simulink library "vmc"  (R2021b)
settings: Solver=VariableStepAuto  StartTime=0.0  StopTime=10.0  RelTol=1e-3
undefined symbols (not defined in the file or in its folder): AVMC_ACCDeltaTqIGain4OVRD_X_kph, AVMC_ACCDeltaTqIGain4OVRD_Y_mps2, AVMC_ACCDeltaTqIGain_X_kph, AVMC_ACCDeltaTqIGain_Y_mps2, AVMC_ACCDeltaTqPGain_X_kph, AVMC_ACCDeltaTqPGain_Y_kph, AVMC_ACCLongSteadyCtrl_X_kph, AVMC_ADSPosGFBDeltaTq_X_kph, AVMC_ADSPosGFBDeltaTq_Y_mps2, AVMC_AggressJerkPCT4AT_X_kph, AVMC_AggressJerkPCT_X_kph, AVMC_AggressLimitPCT4AT_X_kph, AVMC_AggressLimitPCT_X_kph, AVMC_CCLongSteadyCtrl_X_kph, AVMC_DISCDeltaTqIGain_X_kph, AVMC_DISCDeltaTqIGain_Y_mps2, AVMC_DISCDeltaTqPGain_X_kph, AVMC_DISCDeltaTqPGain_Y_kph, AVMC_ESCRegenOut_X_kph, AVMC_ESCRegenOut_Y_Deg, AVMC_ESCRegenOutEnSpd_X_Deg, AVMC_ISOAccLimit_X_mps, AVMC_ISODecLimit_X_mps, AVMC_ISOJerk_X_mps, AVMC_LatESCRegenOut_X_kph, AVMC_LatESCRegenOut_Y_Deg, AVMC_LongAccDeadZone_X_kph, AVMC_LongAccFiltTsforP2_X_Gps, AVMC_MCPresBaseTq_X_bar, AVMC_MSALongSteadyCtrl_X_kph, AVMC_MSAPedalOvrd_X_kph, AVMC_MSASpdBand_X_kph, AVMC_MSATqDownEndTq_X_kph, AVMC_MSATqDownTime_X_kph, AVMC_OPDDisSlideRate_X_Deg, AVMC_OVRD2ActSR2FCMCMD_X_mps2, AVMC_PedalTqRWhlRatio_X_Nm, AVMC_PedalTqRWhlRatio_Y_gps, AVMC_PedalTqRWhlSlipGain_X_rat, AVMC_PedalTqRWhlSlipGain_Y_kph, AVMC_PedalTqRWhSTRGGain_X_deg, AVMC_PedalTqRWhSTRGGain_Y_kph, AVMC_RDCDetectTime_X_kph, AVMC_RDCDetectTime_Y_pct, AVMC_RDCEnSlideRate_X_Deg, AVMC_RearWhlTqRatio_X_Nm, AVMC_RearWhlTqRatio_Y_gps, AVMC_RearWhlTqSlipGain_X_rat, AVMC_RearWhlTqSlipGain_Y_kph, AVMC_RearWhlTqSTRGGain_X_deg, AVMC_RearWhlTqSTRGGain_Y_kph, AVMC_ReqBrkJoinDecSR_X_mps2, AVMC_SoftJerkPCT_X_kph, AVMC_SoftLimitPCT_X_kph, AVMC_StESCYaw_X_kph, AVMC_StESCYaw_Y_Deg, AVMC_StESCYawCom_X_kph, AVMC_StESCYawCom_Y_Gps, AVMC_TMSpdBaseTq_X_rpm, AVMC_VehHoldDecCtrlTime2_X_kph ... (+411)
libraries: hcu_lib x108, simulink x82, tqr x1, simulink_extras x1
(part 6 of 14)

== system vmc/VMC/VMC/ACC_Function/ACC Control Allow Judgement ==
  task_time_s : Inport
  VTQD_ExternalTqAllow_flag : Inport  Port=2
  VTQD_ExtDoorAllow_flg : Inport  Port=3
  AND : Logic  AllPortsSameDT=off  OutDataTypeStr=boolean
  Constant : Constant  Value=KVMC_ExternalTqAllowTime_s
  Constant3 : Constant  Value=TRUE
  Constant4 : Constant  Value=FALSE
  NOT : Logic  Operator=NOT  AllPortsSameDT=off  OutDataTypeStr=boolean
  Relational Operator : RelationalOperator  OutDataTypeStr=boolean  RndMeth=Simplest
  Timer : hcu_lib/Basic_Blocks/Timer
  u2>0 : Switch  Criteria=u2 > Threshold
  VVMC_ACCCtrlAllow_flg : Outport
  wires:
  task_time_s/1 -> [task_time_s]
  Constant/1 -> Relational Operator/2, Timer/4
  VTQD_ExternalTqAllow_flag/1 -> [VTQD_ExternalTqAllow_flag]
  NOT/1 -> Timer/2
  u2>0/1 -> [VVMC_ACCCtrlAllow_flg]  "VVMC_ACCCtrlAllow_flg"
  AND/1 -> NOT/1, Timer/1
  Constant4/1 -> u2>0/3
  Constant3/1 -> u2>0/1
  Timer/1 -> Relational Operator/1
  Relational Operator/1 -> u2>0/2
  [task_time_s] -> Timer/3
  [VVMC_ACCCtrlAllow_flg] -> VVMC_ACCCtrlAllow_flg/1
  [VTQD_ExtDoorAllow_flg] -> AND/2
  [VTQD_ExternalTqAllow_flag] -> AND/1
  VTQD_ExtDoorAllow_flg/1 -> [VTQD_ExtDoorAllow_flg]

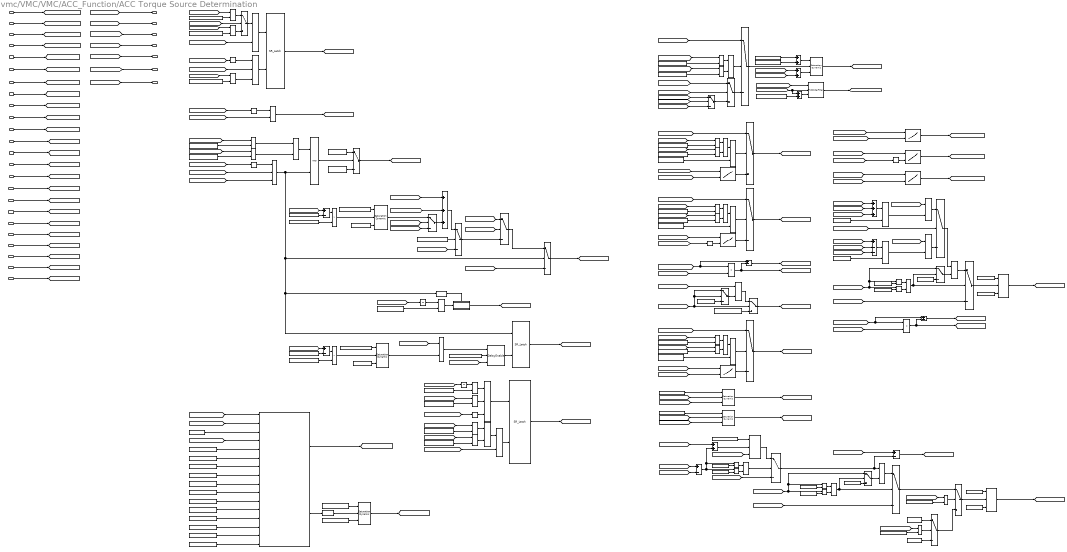
== system vmc/VMC/VMC/ACC_Function/ACC Torque Source Determination ==
  note: TRUE
  VTQD_DriverWhlTqDem_Nm : Inport
  VVMC_ADASWhlTqCal_Nm : Inport  Port=2
  VVMC_FeatArbitrFinal_enum : Inport  Port=3
  VTQD_LowIdleAccPedal_flg : Inport  Port=4
  VINP_ACCObjDist_m : Inport  Port=5
  VINP_TimeGapLevel_enum : Inport  Port=6
  VVMC_ADASActive_flg : Inport  Port=7
  task_time_s : Inport  Port=8
  VINP_LongAccel_Gps : Inport  Port=9
  VINP_VehSpeed_kph : Inport  Port=10
  VVMC_FrRrSlipSpd_kph : Inport  Port=11
  VVMC_CruzWhlTqReq_Nm : Inport  Port=12
  VVMC_CruzActive_flg : Inport  Port=13
  VVMC_MSAWhlTqReq_Nm : Inport  Port=14
  VVMC_MSAActive_flg : Inport  Port=15
  VTQD_RrEDUAvailBrkRgnTq_Nm : Inport  Port=16
  VTQD_FrEDUAvailBrkRgnTq_Nm : Inport  Port=17
  VPMM_DrivetrainSelect_enum : Inport  Port=18
  VINP_SASAngle_Deg : Inport  Port=19
  VDHP_ActAPSPosn_pct : Inport  Port=20
  VTQD_CreepBaseTqD_Nm : Inport  Port=21
  VVMC_ACCVehHoldReqRaw_flg : Inport  Port=22
  VVMC_ADASACCSta_enum : Inport  Port=23
  VTQD_EVDriveMode_enum : Inport  Port=24
  AND{,1,5..6,10,12} (6 alike) : Logic  AllPortsSameDT=off  OutDataTypeStr=boolean
  AND11 : Logic  Inputs=3  AllPortsSameDT=off  OutDataTypeStr=boolean
  AND{2..4,13} (4 alike) : Logic  Operator=OR  AllPortsSameDT=off  OutDataTypeStr=boolean
  Abs : Abs
  Abs1 : Abs
  Add{1,4..6,8,13} (6 alike) : Sum  Inputs=+-
  Add{9..11,28} (4 alike) : Sum
  Add2 : Sum  Inputs=+++
  Add3 : Sum  Inputs=+--
  Add7 : Sum  Inputs=+++
  Cast To Single : DataTypeConversion  OutDataTypeStr=single
  Constant1 : Constant  Value=FALSE
  Constant10 : Constant  Value=ENUM_TIMEGAPLEVEL_LEVEL1
  Constant11 : Constant  Value=ENUM_TIMEGAPLEVEL_LEVEL2
  Constant12 : Constant  Value=ENUM_TIMEGAPLEVEL_LEVEL3
  Constant13 : Constant  Value=ENUM_TIMEGAPLEVEL_LEVEL4
  Constant14 : Constant  Value=KVMC_TimeGapBandLv2_s
  Constant15 : Constant  Value=KVMC_TimeGapBandLv3_s
  Constant16 : Constant  Value=KVMC_TimeGapBandLv4_s
  Constant17 : Constant  Value=TRUE
  Constant18 : Constant  Value=FALSE
  Constant{19,24..26,39,41..46,48,50,52,57,59,65} (17 alike) : Constant  Value=ZERO_FLOAT
  Constant2 : Constant  Value=KTQD_AWDWhlTqRatioSW_flg
  Constant20 : Constant  Value=ENUM_DRIVEMODE_NRM
  Constant208 : Constant  Value=KVMC_ESCLongGBWFilter_raw32
  Constant21 : Constant  Value=KTQD_AWDWhlTqRatioSW_flg
  Constant22 : Constant  Value=ENUM_DRIVEMODE_NRM
  Constant23 : Constant  Value=ENUM_DRIVEMODE_SPORT
  Constant{27..28,37,40,49,51} (6 alike) : Constant  Value=ONE_FLOAT
  Constant29 : Constant  Value=ENUM_FEATARBITRSTA_ACC
  Constant3 : Constant  Value=TRUE
  Constant30 : Constant  Value=ENUM_FEATARBITRSTA_DISC
  Constant31 : Constant  Value=KTQD_RrUppTheldTrq_Nm
  Constant32 : Constant  Value=ENUM_DRIVETRAIN_AWD  VectorParams1D=off  SampleTime=-1
  Constant33 : Constant  Value=KTQD_RrUppTheldTrq_Nm
  Constant34 : Constant  Value=KTQD_RrUppTheldTrq_Nm
  Constant35 : Constant  Value=KTQD_FrUppTheldTrq_Nm
  Constant36 : Constant  Value=KTQD_FrUppTheldTrq_Nm
  Constant38 : Constant  Value=ENUM_DRIVETRAIN_RWD  VectorParams1D=off  SampleTime=-1
  Constant4 : Constant  Value=ENUM_FEATARBITRSTA_ACC
  Constant47 : Constant  Value=KVMC_TimeGapMax_s
  Constant5 : Constant  Value=ENUM_FEATARBITRSTA_DISC
  Constant53 : Constant  Value=KVMC_ACCPedalOvrdPosn_pct
  Constant54 : Constant  Value=KVMC_ACCPedalOvrdResPosn_pct
  Constant58 : Constant  Value=KVMC_ACCPedalOvrdPosn4Hold_pct
  Constant6 : Constant  Value=ENUM_DRIVEMODE_SPORT
  Constant62 : Constant  Value=KVMC_ACCOvrdTestSW_flg
  Constant63 : Constant  Value=KVMC_ACCPedalOvrdPosn_pct
  Constant64 : Constant  Value=KVMC_ACCOvrdPedalTqRatio_Nm
  Constant66 : Constant  Value=KVMC_ACCPedalOvrdRestTime_s
  Constant67 : Constant  Value=KVMC_ACCOvrdPedalTqLinearLim_Nm
  Constant68 : Constant  Value=KVMC_ACCPedalOvrdPosn_pct
  Constant69 : Constant  Value=KVMC_ACCOvrdPedalTqRatio_Nm
  Constant7 : Constant  Value=KVMC_TimeGapMax_s
  Constant71 : Constant  Value=ENUM_ADASACCSTA_STANDBY
  Constant72 : Constant  Value=ENUM_ADASACCSTA_ACTIVE
  Constant73 : Constant  Value=ENUM_ADASACCSTA_ACTIVE
  Constant74 : Constant  Value=ENUM_ADASACCSTA_OVERRIDE
  Constant75 : Constant  Value=KVMC_ACCOvrdPedalTqLinearLim_Nm
  Constant76 : Constant  Value=KTQD_AWDWhlTqRatioSW_flg
  Constant77 : Constant  Value=ENUM_DRIVEMODE_SPORT
  Constant78 : Constant  Value=ENUM_DRIVEMODE_NRM
  Constant8 : Constant  Value=KPH2MPS
  Constant9 : Constant  Value=KVMC_TimeGapBandLv1_s
  DelayEnable1 : hcu_lib/Basic_Blocks/DelayEnable
  Detect Increase : simulink/Logic and Bit Operations/Detect Increase  vinit=0.0  OutDataTypeStr=boolean
  Divide{,3,5,7} (4 alike) : Product  Inputs=**
  Divide1 : Product  Inputs=*/
  Divide2 : Product  Inputs=*/
  Divide4 : Product  Inputs=*/
  Equal{1..8} (8 alike) : RelationalOperator  Operator===  OutDataTypeStr=boolean  RndMeth=Simplest
  FirstOrderFilter6 : hcu_lib/Basic_Blocks/FirstOrderFilter
  Logical Operator1 : Logic  Inputs=3  AllPortsSameDT=off  OutDataTypeStr=boolean
  Logical Operator2 : Logic  Operator=OR  AllPortsSameDT=off  OutDataTypeStr=boolean
  Logical Operator4 : Logic  AllPortsSameDT=off  OutDataTypeStr=boolean
  Logical Operator5 : Logic  Operator=OR  AllPortsSameDT=off  OutDataTypeStr=boolean
  MMAP_PedalTqRWhlSlipGain_Z_Nm : Lookup_n-D  BreakpointsForDimension1=AVMC_PedalTqRWhlSlipGain_Y_kph  BreakpointsForDimension2=AVMC_PedalTqRWhlSlipGain_X_rat  Table=MVMC_PedalTqRWhlSlipGain_Z_Nm  InternalRulePriority=Speed  RndMeth=Simplest  InputSameDT=on
      settings: InputPortMap=u0,u1
  MMAP_RearWhlTqSlipGain_Z_Nm : Lookup_n-D  BreakpointsForDimension1=AVMC_RearWhlTqSlipGain_Y_kph  BreakpointsForDimension2=AVMC_RearWhlTqSlipGain_X_rat  Table=MVMC_RearWhlTqSlipGain_Z_Nm  InternalRulePriority=Speed  RndMeth=Simplest  InputSameDT=on
      settings: InputPortMap=u0,u1
  MVMC_PedalTqRWhSTRGGain_Z_Nm : Lookup_n-D  BreakpointsForDimension1=AVMC_PedalTqRWhSTRGGain_Y_kph  BreakpointsForDimension2=AVMC_PedalTqRWhSTRGGain_X_deg  Table=MVMC_PedalTqRWhSTRGGain_Z_Nm  InternalRulePriority=Speed  RndMeth=Simplest  InputSameDT=on
      settings: InputPortMap=u0,u1
  MVMC_PedalTqRWhlRatio_Z_rat : Lookup_n-D  BreakpointsForDimension1=AVMC_PedalTqRWhlRatio_Y_gps  BreakpointsForDimension2=AVMC_PedalTqRWhlRatio_X_Nm  Table=MVMC_PedalTqRWhlRatio_Z_rat  InternalRulePriority=Speed  RndMeth=Simplest  InputSameDT=on
      settings: InputPortMap=u0,u1
  MVMC_RearWhlTqRatio_Z_rat : Lookup_n-D  BreakpointsForDimension1=AVMC_RearWhlTqRatio_Y_gps  BreakpointsForDimension2=AVMC_RearWhlTqRatio_X_Nm  Table=MVMC_RearWhlTqRatio_Z_rat  InternalRulePriority=Speed  RndMeth=Simplest  InputSameDT=on
      settings: InputPortMap=u0,u1
  MVMC_RearWhlTqSTRGGain_Z_Nm : Lookup_n-D  BreakpointsForDimension1=AVMC_RearWhlTqSTRGGain_Y_kph  BreakpointsForDimension2=AVMC_RearWhlTqSTRGGain_X_deg  Table=MVMC_RearWhlTqSTRGGain_Z_Nm  InternalRulePriority=Speed  RndMeth=Simplest  InputSameDT=on
      settings: InputPortMap=u0,u1
  Max : MinMax  Function=max  Inputs=2
  Max1 : MinMax  Inputs=2
  Max2 : MinMax  Inputs=2
  Max3 : MinMax  Function=max  Inputs=2
  Min : MinMax  Function=max  Inputs=2
  NOT{,3,5,7} (4 alike) : Logic  Operator=NOT  AllPortsSameDT=off  OutDataTypeStr=boolean
  OR1 : Logic  Operator=OR  Inputs=3  AllPortsSameDT=off  OutDataTypeStr=boolean
  OR2 : Logic  Operator=OR  AllPortsSameDT=off  OutDataTypeStr=boolean
  OR3 : Logic  Operator=OR  AllPortsSameDT=off  OutDataTypeStr=boolean
  OR4 : Logic  Operator=OR  AllPortsSameDT=off  OutDataTypeStr=boolean
  Relational Operator{,11,13,19} (4 alike) : RelationalOperator  Operator=>  OutDataTypeStr=boolean  RndMeth=Simplest
  Relational Operator{10,12,14,16} (4 alike) : RelationalOperator  Operator=<  OutDataTypeStr=boolean  RndMeth=Simplest
  Relational Operator15 : RelationalOperator  OutDataTypeStr=boolean  RndMeth=Simplest
  Relational Operator17 : RelationalOperator  OutDataTypeStr=boolean  RndMeth=Simplest
  Relational Operator{2..3,5,9,21..22} (6 alike) : RelationalOperator  Operator===  OutDataTypeStr=boolean  RndMeth=Simplest
  Relational Operator23 : RelationalOperator  Operator=~=  OutDataTypeStr=boolean  RndMeth=Simplest
  Relational Operator24 : RelationalOperator  Operator=~=  OutDataTypeStr=boolean  RndMeth=Simplest
  SR_Latch : hcu_lib/Basic_Blocks/SR_Latch
  SR_Latch1 : hcu_lib/Basic_Blocks/SR_Latch
  SR_Latch2 : hcu_lib/Basic_Blocks/SR_Latch
  Saturation Dynamic{,1..8} (9 alike) : simulink/Discontinuities/Saturation Dynamic  OutMin=[]  OutMax=[]  OutDataTypeStr=Inherit: Same as second input  OutDataType=fixdt(1, 16)  OutScaling=2^-10  DoSatur=off
  Switch{,4..7,9..10,12,14..17} (12 alike) : Switch  Criteria=u2 > Threshold
  Switch{1,3,8,11,13} (5 alike) : Switch  Criteria=u2 ~= 0
  Switch2 : Switch
  TimeGapJudgement : Stateflow chart  TreatAsAtomicUnit=on
  Triggered Subsystem2 : Subsystem  TreatAsAtomicUnit=on
  Unit Delay : UnitDelay  SampleTime=-1  HasFrameUpgradeWarning=on
  Unit Delay1 : UnitDelay  SampleTime=-1  HasFrameUpgradeWarning=on
  u2 > 0 : Switch  Criteria=u2 > Threshold
  u2 > 0 (1) : Switch  Criteria=u2 > Threshold
  u2 > 0 (1)1 : Switch  Criteria=u2 > Threshold
  u2 > 0 (1)2 : Switch  Criteria=u2 > Threshold
  VVMC_ACCPedalOvrd_flg : Outport
  VVMC_ADASWhlTqReq_Nm : Outport  Port=2
  VVMC_TimeGapCalcu_s : Outport  Port=3
  VVMC_AccPedalOvrdDISC_flg : Outport  Port=4
  VVMC_RearTqRatio_rat : Outport  Port=5
  VVMC_TimeGapJudge_flag : Outport  Port=6
  VVMC_ACCOvrdMemTq_Nm : Outport  Port=7
  wires:
  [VVMC_ACCPedalTqEnOvrd_flg] -> Logical Operator1/2
  SR_Latch/1 -> [VVMC_ACCPedalTqEnOvrd_flg]  "VVMC_ACCPedalTqEnOvrd_flg"
  VVMC_ADASActive_flg/1 -> [VVMC_ADASActive_flg]
  Saturation Dynamic2/1 -> [VVMC_TimeGapCalcu_s]  "VVMC_TimeGapCalcu_s"
  [VVMC_TimeGapCalcu_s] -> VVMC_TimeGapCalcu_s/1
  TimeGapJudgement/2(VVMC_TimeGapCalcu_s) -> Cast To Single/1
  Constant7/1 -> TimeGapJudgement/16(KVMC_TimeGapMax_s)
  Constant19/1 -> TimeGapJudgement/15(ZERO_FLOAT)
  Constant18/1 -> TimeGapJudgement/14(FALSE)
  Constant17/1 -> TimeGapJudgement/13(TRUE)
  Constant16/1 -> TimeGapJudgement/12(KVMC_TimeGapBandLv4_s)
  Constant13/1 -> TimeGapJudgement/11(ENUM_TIMEGAPLEVEL_LEVEL4)
  Constant15/1 -> TimeGapJudgement/10(KVMC_TimeGapBandLv3_s)
  Constant12/1 -> TimeGapJudgement/9(ENUM_TIMEGAPLEVEL_LEVEL3)
  Constant14/1 -> TimeGapJudgement/8(KVMC_TimeGapBandLv2_s)
  Constant11/1 -> TimeGapJudgement/7(ENUM_TIMEGAPLEVEL_LEVEL2)
  Constant9/1 -> TimeGapJudgement/6(KVMC_TimeGapBandLv1_s)
  Constant10/1 -> TimeGapJudgement/5(ENUM_TIMEGAPLEVEL_LEVEL1)
  TimeGapJudgement/1(VVMC_TimeGapJudge_flag) -> [VVMC_TimeGapJudge_flag]  "VVMC_TimeGapJudge_flag"
  [VINP_ACCObjDist_m] -> TimeGapJudgement/1(VINP_ACCObjDist_m)
  [VINP_VehSpeed_kph] -> TimeGapJudgement/2(VINP_VehSpeed_kph)
  Constant8/1 -> TimeGapJudgement/3(KPH2MPS)
  [VINP_TimeGapLevel_enum] -> TimeGapJudgement/4(VINP_TimeGapLevel_enum)
  VINP_TimeGapLevel_enum/1 -> [VINP_TimeGapLevel_enum]
  VINP_ACCObjDist_m/1 -> [VINP_ACCObjDist_m]
  Logical Operator2/1 -> AND/1
  Relational Operator3/1 -> Logical Operator2/2
  Constant5/1 -> Relational Operator3/2
  [VVMC_FeatArbitrFinal_enum] -> Relational Operator3/1
  Logical Operator1/1 -> SR_Latch1/1, Detect Increase/1, u2 > 0 (1)/2, AND/2
  Constant4/1 -> Relational Operator2/2
  [VVMC_FeatArbitrFinal_enum] -> Relational Operator2/1
  VTQD_DriverWhlTqDem_Nm/1 -> [VTQD_DriverWhlTqDem_Nm]
  VVMC_ADASWhlTqCal_Nm/1 -> [VVMC_ADASWhlTqCal_Nm]
  [VVMC_ACCPedalOvrd_flg] -> VVMC_ACCPedalOvrd_flg/1
  [VVMC_ADASWhlTqReq_Nm] -> VVMC_ADASWhlTqReq_Nm/1
  u2 > 0 (1)/1 -> [VVMC_ADASWhlTqReq_Nm]  "VVMC_ADASWhlTqReq_Nm"
  [VVMC_ADASWhlTqCal_Nm] -> u2 > 0 (1)/3
  Constant1/1 -> u2 > 0/3
  Constant3/1 -> u2 > 0/1
  u2 > 0/1 -> [VVMC_ACCPedalOvrd_flg]  "VVMC_ACCPedalOvrd_flg"
  AND/1 -> u2 > 0/2
  Relational Operator2/1 -> Logical Operator2/1
  VVMC_FeatArbitrFinal_enum/1 -> [VVMC_FeatArbitrFinal_enum]
  VTQD_LowIdleAccPedal_flg/1 -> [VTQD_LowIdleAccPedal_flg]
  NOT/1 -> Logical Operator1/1
  [VTQD_LowIdleAccPedal_flg] -> NOT/1
  [VVMC_AccPedalOvrdDISC_flg] -> VVMC_AccPedalOvrdDISC_flg/1
  Logical Operator4/1 -> [VVMC_AccPedalOvrdDISC_flg]  "VVMC_AccPedalOvrdDISC_flg"
  NOT3/1 -> Logical Operator4/1
  [VVMC_ACCPedalTqEnOvrd_flg] -> Logical Operator4/2
  [VTQD_LowIdleAccPedal_flg] -> NOT3/1
  [VTQD_LowIdleAccPedal_flg] -> OR1/2
  OR1/1 -> SR_Latch/2
  task_time_s/1 -> [task_time_s]
  [VVMC_VMCWhlTq4RatioCalcu_Nm] -> MVMC_RearWhlTqRatio_Z_rat/2
  VINP_LongAccel_Gps/1 -> [VINP_LongAccel_Gps]
  [VVMC_ESCLongAccelFilt_Gps] -> MVMC_RearWhlTqRatio_Z_rat/1
  Switch17/1 -> [VVMC_RearTqRatioBfrSlip_rat]  "VVMC_RearTqRatioBfrSlip_rat"
  [VVMC_RearTqRatio_rat] -> VVMC_RearTqRatio_rat/1
  VINP_VehSpeed_kph/1 -> [VINP_VehSpeed_kph]
  VVMC_FrRrSlipSpd_kph/1 -> [VVMC_FrRrSlipSpd_kph]
  [VVMC_VMCWhlTq4RatioCalcu_Nm] -> Divide/1, Add1/1
  [VVMC_RearTqRatioBfrSlip_rat] -> Divide/2
  Divide/1 -> [VVMC_ADASRrWhlTqBfrSlip_Nm], Add1/2  "VVMC_ADASRrWhlTqBfrSlip_Nm"
  Add1/1 -> [VVMC_ADASFrWhlTqBfrSlip_Nm]  "VVMC_ADASFrWhlTqBfrSlip_Nm"
  [VINP_VehSpeed_kph] -> Switch/2, Switch4/2, Switch4/1
  Constant24/1 -> Switch/3
  Divide1/1 -> Switch/1
  [VVMC_FrRrSlipSpd_kph] -> Divide1/1
  Switch/1 -> [VVMC_FrRrSlipRate_rat]  "VVMC_FrRrSlipRate_rat"
  [VVMC_FrRrSlipRate_rat] -> MMAP_RearWhlTqSlipGain_Z_Nm/2
  [VINP_VehSpeed_kph] -> MMAP_RearWhlTqSlipGain_Z_Nm/1
  Switch14/1 -> [VVMC_RearWhlTqSlipGain_Nm]  "VVMC_RearWhlTqSlipGain_Nm"
  [VVMC_RearTqRatioBfrSlip_rat] -> Switch1/3
  Saturation Dynamic5/1 -> [VVMC_RearTqRatioAftSlip_rat]  "VVMC_RearTqRatioAftSlip_rat"
  Switch2/1 -> Divide2/1
  Divide2/1 -> Switch1/1
  Constant27/1 -> Switch3/3
  Switch3/1 -> Divide2/2
  Constant28/1 -> Switch4/3
  Switch4/1 -> Divide1/2
  [VVMC_ADASActive_flg] -> Logical Operator1/3
  Relational Operator5/1 -> Logical Operator5/1
  Relational Operator9/1 -> Logical Operator5/2
  [VVMC_FeatArbitrFinal_enum] -> Relational Operator5/1
  Constant30/1 -> Relational Operator9/2
  [VVMC_FeatArbitrFinal_enum] -> Relational Operator9/1
  Constant29/1 -> Relational Operator5/2
  Logical Operator5/1 -> Switch5/2
  [VTQD_DriverWhlTqDem_Nm] -> Switch7/3
  [VVMC_ADASWhlTqReq_Nm] -> Switch5/1
  Saturation Dynamic4/1 -> [VVMC_VMCWhlTq4RatioCalcu_Nm]  "VVMC_VMCWhlTq4RatioCalcu_Nm"
  VVMC_MSAActive_flg/1 -> [VVMC_MSAActive_flg]
  VVMC_MSAWhlTqReq_Nm/1 -> [VVMC_MSAWhlTqReq_Nm]
  VVMC_CruzWhlTqReq_Nm/1 -> [VVMC_CruzWhlTqReq_Nm]
  VVMC_CruzActive_flg/1 -> [VVMC_CruzActive_flg]
  [VVMC_CruzActive_flg] -> Switch6/2
  [VVMC_CruzWhlTqReq_Nm] -> Switch6/1
  Switch6/1 -> Switch5/3
  [VVMC_MSAActive_flg] -> Switch7/2
  [VVMC_MSAWhlTqReq_Nm] -> Switch7/1
  Switch7/1 -> Switch6/3
  Add4/1 -> [VVMC_ADASFrWhlTqAftSlip_Nm]  "VVMC_ADASFrWhlTqAftSlip_Nm"
  Divide3/1 -> Add4/2, [VVMC_ADASRrWhlTqAftSlip_Nm]  "VVMC_ADASRrWhlTqAftSlip_Nm"
  [VVMC_RearTqRatioAftSlip_rat] -> Divide3/2
  [VVMC_VMCWhlTq4RatioCalcu_Nm] -> Add4/1, Divide3/1
  VTQD_FrEDUAvailBrkRgnTq_Nm/1 -> [VTQD_FrEDUAvailBrkRgnTq_Nm]
  VTQD_RrEDUAvailBrkRgnTq_Nm/1 -> [VTQD_RrEDUAvailBrkRgnTq_Nm]
  [VVMC_ADASFrWhlTqAftSlip_Nm] -> Saturation Dynamic/2
  Constant35/1 -> Saturation Dynamic/1
  [VTQD_FrEDUAvailBrkRgnTq_Nm] -> Saturation Dynamic/3
  Constant31/1 -> Saturation Dynamic1/1
  [VVMC_ADASRrWhlTqAftSlip_Nm] -> Saturation Dynamic1/2
  [VTQD_RrEDUAvailBrkRgnTq_Nm] -> Saturation Dynamic1/3
  Saturation Dynamic/1 -> [VVMC_ADASFrWhlTqAftLim_Nm]  "VVMC_ADASFrWhlTqAftLim_Nm"
  Saturation Dynamic1/1 -> [VVMC_ADASRrWhlTqAftLim_Nm]  "VVMC_ADASRrWhlTqAftLim_Nm"
  [VVMC_ADASFrWhlTqAftSlip_Nm] -> Add5/1
  [VVMC_ADASFrWhlTqAftLim_Nm] -> Add5/2
  [VVMC_ADASRrWhlTqAftLim_Nm] -> Switch8/3
  Saturation Dynamic3/1 -> Switch8/1
  [VVMC_ADASRrWhlTqAftLim_Nm] -> Add9/1
  Constant33/1 -> Saturation Dynamic3/1
  [VTQD_RrEDUAvailBrkRgnTq_Nm] -> Saturation Dynamic3/3
  Add9/1 -> Saturation Dynamic3/2
  Switch13/1 -> Divide4/2
  Constant37/1 -> Switch13/3
  Divide4/1 -> Switch11/1
  Switch8/1 -> Add6/2, Divide4/1  "VVMC_ADASRrWhlTq_Nm"
  Saturation Dynamic6/1 -> [VVMC_RearTqRatio_rat]  "VVMC_RearTqRatio_rat"
  [VVMC_RearTqRatioBfrSlip_rat] -> Switch11/3
  [VTQD_RrEDUAvailBrkRgnTq_Nm] -> Add11/2
  Constant34/1 -> Add10/2
  [VTQD_FrEDUAvailBrkRgnTq_Nm] -> Add11/1
  Constant36/1 -> Add10/1
  Add10/1 -> Saturation Dynamic4/1
  Add11/1 -> Saturation Dynamic4/3
  Switch5/1 -> Saturation Dynamic4/2
  [VVMC_VMCWhlTq4RatioCalcu_Nm] -> Add6/1
  Add6/1 -> [VVMC_ADASFrWhlTq_Nm]  "VVMC_ADASFrWhlTq_Nm"
  VPMM_DrivetrainSelect_enum/1 -> [VPMM_DrivetrainSelect_enum]
  [VPMM_DrivetrainSelect_enum] -> Equal3/1
  Constant32/1 -> Equal3/2
  Switch11/1 -> Switch9/1
  Equal3/1 -> Switch9/2
  Constant38/1 -> Equal1/2
  [VPMM_DrivetrainSelect_enum] -> Equal1/1
  Equal1/1 -> Switch10/2
  Switch10/1 -> Switch9/3
  Constant39/1 -> Switch10/3
  Constant40/1 -> Switch10/1
  Constant42/1 -> Relational Operator10/2
  Relational Operator/1 -> AND2/1
  Relational Operator10/1 -> AND2/2
  Constant41/1 -> Relational Operator/2
  [VVMC_VMCWhlTq4RatioCalcu_Nm] -> Relational Operator10/1, Switch3/1, Relational Operator/1
  AND2/1 -> Switch3/2, Switch1/2
  Constant44/1 -> Relational Operator12/2
  Relational Operator11/1 -> AND3/1
  Relational Operator12/1 -> AND3/2
  Constant43/1 -> Relational Operator11/2
  Add5/1 -> Relational Operator11/1, Add9/2, Relational Operator12/1
  AND3/1 -> Switch8/2
  Constant46/1 -> Relational Operator14/2
  Relational Operator13/1 -> AND4/1
  Relational Operator14/1 -> AND4/2
  Constant45/1 -> Relational Operator13/2
  [VVMC_VMCWhlTq4RatioCalcu_Nm] -> Relational Operator14/1, Switch13/1, Relational Operator13/1
  AND4/1 -> Switch13/2, Switch11/2
  Cast To Single/1 -> Saturation Dynamic2/2
  Constant47/1 -> Saturation Dynamic2/1
  Constant48/1 -> Saturation Dynamic2/3
  [VVMC_TimeGapJudge_flag] -> VVMC_TimeGapJudge_flag/1
  Abs/1 -> MVMC_RearWhlTqSTRGGain_Z_Nm/2
  [VINP_VehSpeed_kph] -> MVMC_RearWhlTqSTRGGain_Z_Nm/1
  [VINP_SASAngle_Deg] -> Abs/1
  Switch16/1 -> [VVMC_RearWhlTqSTRGGain_Nm]  "VVMC_RearWhlTqSTRGGain_Nm"
  [VVMC_RearWhlTqSTRGGain_Nm] -> Add2/3
  [VVMC_RearWhlTqSTRGGain_Nm] -> Add3/3
  [VVMC_ADASRrWhlTqBfrSlip_Nm] -> Add2/1
  [VVMC_RearWhlTqSlipGain_Nm] -> Add3/2
  Max1/1 -> Max3/2
  Add2/1 -> Max/1
  [VVMC_VMCWhlTq4RatioCalcu_Nm] -> Switch2/2
  [VVMC_RearWhlTqSlipGain_Nm] -> Add2/2
  Constant25/1 -> Max/2
  Add3/1 -> Max1/1
  Constant26/1 -> Max1/2
  [VVMC_ADASRrWhlTqBfrSlip_Nm] -> Add3/1
  Max/1 -> Max2/2
  VINP_SASAngle_Deg/1 -> [VINP_SASAngle_Deg]
  [VVMC_VMCWhlTq4RatioCalcu_Nm] -> Max2/1
  Max2/1 -> Switch2/1
  [VVMC_VMCWhlTq4RatioCalcu_Nm] -> Max3/1
  Max3/1 -> Switch2/3
  Constant49/1 -> Saturation Dynamic5/1
  Switch1/1 -> Saturation Dynamic5/2
  Constant50/1 -> Saturation Dynamic5/3
  Constant52/1 -> Saturation Dynamic6/3
  Switch9/1 -> Saturation Dynamic6/2
  Constant51/1 -> Saturation Dynamic6/1
  [VDHP_ActAPSPosn_pct] -> Relational Operator15/1
  Relational Operator15/1 -> Switch12/3
  AND5/1 -> SR_Latch/1
  Constant53/1 -> Relational Operator15/2
  VDHP_ActAPSPosn_pct/1 -> [VDHP_ActAPSPosn_pct]
  VTQD_CreepBaseTqD_Nm/1 -> [VTQD_CreepBaseTqD_Nm]
  [VTQD_CreepBaseTqD_Nm] -> Add7/2
  Switch15/1 -> Add7/3
  Triggered Subsystem2/1(Out1) -> [VVMC_ACCOvrdMemTq_Nm]  "VVMC_ACCOvrdMemTq_Nm"
  Unit Delay/1 -> Min/1
  [VVMC_ADASWhlTqReq_Nm] -> Unit Delay/1
  Add7/1 -> u2 > 0 (1)1/1
  [VVMC_ACCOvrdMemTq_Nm] -> Add7/1
  Detect Increase/1 -> Triggered Subsystem2/Trigger
  Min/1 -> Triggered Subsystem2/1(In1)
  Constant57/1 -> Min/2
  [VVMC_ACCOvrdMemTq_Nm] -> VVMC_ACCOvrdMemTq_Nm/1
  VVMC_ACCVehHoldReqRaw_flg/1 -> [VVMC_ACCVehHoldReqRaw_flg]
  [VVMC_ACCVehHoldReqRaw_flg] -> Switch12/2
  Switch12/1 -> AND5/1
  Constant58/1 -> Relational Operator17/2
  [VDHP_ActAPSPosn_pct] -> Relational Operator17/1
  Relational Operator17/1 -> Switch12/1
  Relational Operator16/1 -> OR1/3
  [VDHP_ActAPSPosn_pct] -> Add8/1
  Constant63/1 -> Add8/2
  Add8/1 -> Divide5/1
  Constant64/1 -> Divide5/2
  [VTQD_DriverWhlTqDem_Nm] -> Relational Operator19/1
  Saturation Dynamic8/1 -> Relational Operator19/2
  Relational Operator19/1 -> DelayEnable1/1
  SR_Latch1/1 -> [VVMC_ACCOvrdBackDrTq_flg]  "VVMC_ACCOvrdBackDrTq_flg"
  [VVMC_ACCOvrdBackDrTq_flg] -> Switch15/2
  Divide5/1 -> Saturation Dynamic7/2
  [VTQD_DriverWhlTqDem_Nm] -> Switch15/3
  Constant66/1 -> DelayEnable1/2
  [task_time_s] -> DelayEnable1/3
  DelayEnable1/1 -> SR_Latch1/2
  Saturation Dynamic7/1 -> Switch15/1  "VVMC_ADASOvrdWhlTqCtrl_Nm"
  Constant69/1 -> Divide7/2
  Add13/1 -> Divide7/1
  Constant68/1 -> Add13/2
  [VDHP_ActAPSPosn_pct] -> Add13/1
  Constant62/1 -> u2 > 0 (1)1/2
  [VTQD_DriverWhlTqDem_Nm] -> u2 > 0 (1)1/3
  u2 > 0 (1)1/1 -> u2 > 0 (1)2/3  "VVMC_ADASOvrdWhlTq_Nm"
  VVMC_ADASACCSta_enum/1 -> [VVMC_ADASACCSta_enum]
  [VVMC_ADASACCSta_enum] -> Unit Delay1/1
  Unit Delay1/1 -> Relational Operator21/1
  Constant71/1 -> Relational Operator21/2
  Constant72/1 -> Relational Operator22/2
  [VVMC_ADASACCSta_enum] -> Relational Operator22/1
  [VTQD_LowIdleAccPedal_flg] -> NOT5/1
  Relational Operator22/1 -> AND11/2
  Relational Operator21/1 -> AND11/1
  NOT5/1 -> AND11/3
  AND11/1 -> SR_Latch2/1
  SR_Latch2/1 -> [VVMC_ACCActivePedalOn_flg]  "VVMC_ACCActivePedalOn_flg"
  [VTQD_LowIdleAccPedal_flg] -> AND13/2
  [VVMC_ADASACCSta_enum] -> Relational Operator23/1
  Constant73/1 -> Relational Operator23/2
  Constant74/1 -> Relational Operator24/2
  [VVMC_ADASACCSta_enum] -> Relational Operator24/1
  Relational Operator23/1 -> AND12/1
  Relational Operator24/1 -> AND12/2
  AND12/1 -> AND13/1
  AND13/1 -> SR_Latch2/2
  [VVMC_ACCActivePedalOn_flg] -> u2 > 0 (1)2/2
  [VTQD_DriverWhlTqDem_Nm] -> u2 > 0 (1)2/1
  u2 > 0 (1)2/1 -> u2 > 0 (1)/1  "VVMC_ADASWhlTqReqOvrd_Nm"
  [VDHP_ActAPSPosn_pct] -> Relational Operator16/1
  Constant54/1 -> Relational Operator16/2
  Constant59/1 -> Saturation Dynamic7/3
  Constant75/1 -> Saturation Dynamic7/1
  Constant67/1 -> Saturation Dynamic8/1
  Constant65/1 -> Saturation Dynamic8/3
  Divide7/1 -> Saturation Dynamic8/2
  [VVMC_ADASActive_flg] -> AND5/2
  [VVMC_ADASActive_flg] -> NOT7/1
  NOT7/1 -> OR1/1
  Constant208/1 -> Add28/2
  Add28/1 -> FirstOrderFilter6/3
  [task_time_s] -> Add28/1, FirstOrderFilter6/2
  [VINP_LongAccel_Gps] -> FirstOrderFilter6/1
  FirstOrderFilter6/1 -> [VVMC_ESCLongAccelFilt_Gps]  "VVMC_ESCLongAccelFilt_Gps"
  [VTQD_EVDriveMode_enum] -> Equal4/1
  OR2/1 -> AND10/1
  AND10/1 -> Switch14/2
  Equal5/1 -> OR2/2
  [VVMC_PedalTqRWhlSlipGain_Nm] -> Switch14/1
  Constant77/1 -> Equal4/2
  [VTQD_EVDriveMode_enum] -> Equal5/1
  Constant76/1 -> AND10/2
  Constant78/1 -> Equal5/2
  Equal4/1 -> OR2/1
  MMAP_RearWhlTqSlipGain_Z_Nm/1 -> Switch14/3
  [VTQD_EVDriveMode_enum] -> Equal2/1
  OR3/1 -> AND1/1
  Equal6/1 -> OR3/2
  Equal2/1 -> OR3/1
  Constant20/1 -> Equal6/2
  Constant2/1 -> AND1/2
  [VTQD_EVDriveMode_enum] -> Equal6/1
  [VVMC_PedalTqRWhSTRGGain_Nm] -> Switch16/1
  Constant6/1 -> Equal2/2
  AND1/1 -> Switch16/2
  MVMC_RearWhlTqSTRGGain_Z_Nm/1 -> Switch16/3
  AND6/1 -> Switch17/2
  Constant23/1 -> Equal7/2
  [VVMC_PedalTqRWhlRatio_rat] -> Switch17/1
  [VTQD_EVDriveMode_enum] -> Equal8/1
  Constant21/1 -> AND6/2
  Constant22/1 -> Equal8/2
  Equal7/1 -> OR4/1
  Equal8/1 -> OR4/2
  OR4/1 -> AND6/1
  [VTQD_EVDriveMode_enum] -> Equal7/1
  MVMC_RearWhlTqRatio_Z_rat/1 -> Switch17/3
  [VVMC_FrRrSlipRate_rat] -> MMAP_PedalTqRWhlSlipGain_Z_Nm/2
  [VVMC_VMCWhlTq4RatioCalcu_Nm] -> MVMC_PedalTqRWhlRatio_Z_rat/2
  MVMC_PedalTqRWhlRatio_Z_rat/1 -> [VVMC_PedalTqRWhlRatio_rat]  "VVMC_PedalTqRWhlRatio_rat"
  MVMC_PedalTqRWhSTRGGain_Z_Nm/1 -> [VVMC_PedalTqRWhSTRGGain_Nm]  "VVMC_PedalTqRWhSTRGGain_Nm"
  [VINP_VehSpeed_kph] -> MMAP_PedalTqRWhlSlipGain_Z_Nm/1
  [VVMC_ESCLongAccelFilt_Gps] -> MVMC_PedalTqRWhlRatio_Z_rat/1
  MMAP_PedalTqRWhlSlipGain_Z_Nm/1 -> [VVMC_PedalTqRWhlSlipGain_Nm]  "VVMC_PedalTqRWhlSlipGain_Nm"
  Abs1/1 -> MVMC_PedalTqRWhSTRGGain_Z_Nm/2
  [VINP_VehSpeed_kph] -> MVMC_PedalTqRWhSTRGGain_Z_Nm/1
  [VINP_SASAngle_Deg] -> Abs1/1
  VTQD_EVDriveMode_enum/1 -> [VTQD_EVDriveMode_enum]

== system vmc/VMC/VMC/ACC_Function/Hand Shaking ==
  VVMC_FeatArbitrFinal_enum : Inport
  VVMC_ACCCtrlAllow_flg : Inport  Port=2
  VVMC_ACCShutOffHold_flg : Inport  Port=3
  VINP_ADASACCSta_enum : Inport  Port=4
  Constant1 : Constant  Value=TRUE
  Constant2 : Constant  Value=ENUM_FEATARBITRSTA_DISC
  Constant3 : Constant  Value=FALSE
  Constant4 : Constant  Value=ENUM_FEATARBITRSTA_ACC
  Constant5 : Constant  Value=TRUE
  Constant6 : Constant  Value=FALSE
  Constant7 : Constant  Value=ENUM_FEATARBITRSTA_AEB
  Constant9 : Constant  Value=ENUM_ADASACCSTA_ACTIVE
  Logical Operator : Logic  AllPortsSameDT=off  OutDataTypeStr=boolean
  Logical Operator1 : Logic  Operator=OR  Inputs=4  AllPortsSameDT=off  OutDataTypeStr=boolean
  OR1 : Logic  AllPortsSameDT=off  OutDataTypeStr=boolean
  Relational Operator{1..3,6} (4 alike) : RelationalOperator  Operator===  OutDataTypeStr=boolean  RndMeth=Simplest
  Switch : Switch  Criteria=u2 > Threshold
  u2>0 : Switch  Criteria=u2 > Threshold
  VVMC_ACCCtrlAvail_flg : Outport
  VVMC_ADASActive_flg : Outport  Port=2
  wires:
  Logical Operator1/1 -> Logical Operator/1
  Relational Operator2/1 -> Logical Operator1/3
  Constant4/1 -> Relational Operator2/2
  [VVMC_FeatArbitrFinal_enum] -> Relational Operator2/1
  [VVMC_ACCCtrlAvail_flg] -> VVMC_ACCCtrlAvail_flg/1
  VVMC_FeatArbitrFinal_enum/1 -> [VVMC_FeatArbitrFinal_enum]
  [VVMC_FeatArbitrFinal_enum] -> Relational Operator1/1
  Constant2/1 -> Relational Operator1/2
  [VVMC_ADASActive_flg] -> VVMC_ADASActive_flg/1
  [VVMC_ACCCtrlAllow_flg] -> Switch/2, Logical Operator/2
  Switch/1 -> [VVMC_ACCCtrlAvail_flg]  "VVMC_ACCCtrlAvail_flg"
  Constant6/1 -> Switch/3
  Constant5/1 -> Switch/1
  VVMC_ACCCtrlAllow_flg/1 -> [VVMC_ACCCtrlAllow_flg]
  Relational Operator1/1 -> Logical Operator1/4
  Logical Operator/1 -> u2>0/2
  Constant1/1 -> u2>0/1
  u2>0/1 -> [VVMC_ADASActive_flg]  "VVMC_ADASActive_flg"
  Constant3/1 -> u2>0/3
  VVMC_ACCShutOffHold_flg/1 -> [VVMC_ACCShutOffHold_flg]
  [VVMC_ACCShutOffHold_flg] -> Logical Operator1/2
  [VINP_ADASACCSta_enum] -> Relational Operator3/1
  Constant9/1 -> Relational Operator3/2
  OR1/1 -> Logical Operator1/1
  VINP_ADASACCSta_enum/1 -> [VINP_ADASACCSta_enum]
  Relational Operator3/1 -> OR1/1
  [VVMC_FeatArbitrFinal_enum] -> Relational Operator6/1
  Constant7/1 -> Relational Operator6/2
  Relational Operator6/1 -> OR1/2
